simulink model "ccf"  (R2015b)
settings: Solver=VariableStepAuto  StartTime=0.0  StopTime=10.0  RelTol=1e-3
values from neighbouring files (symbols this model uses):
  Fx = inv((C*inv(-Ar)*B(:,1)))    [untitled.m]
settings Model: Creator=ovi  LastModifiedBy=ovi

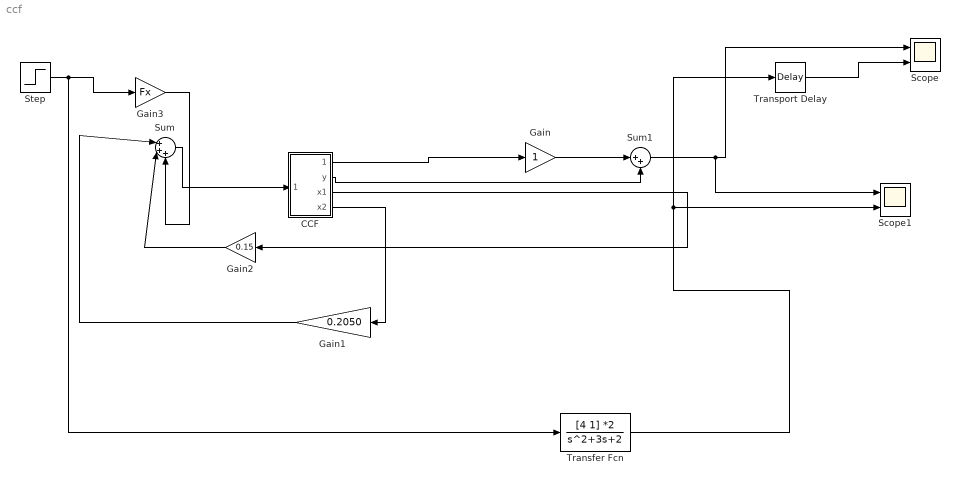
== system ccf ==
  CCF : Subsystem
  Gain : Gain
  Gain1 : Gain  Gain=0.2050
  Gain2 : Gain  Gain=0.15
  Gain3 : Gain  Gain=Fx
  Scope : Scope  NumInputPorts=2
  Scope1 : Scope  NumInputPorts=2
  Step : Step  SampleTime=0
  Sum : Sum  Inputs=|+++
  Sum1 : Sum  Inputs=|++
  Transfer Fcn : TransferFcn  Numerator=[4 1] *2  Denominator=[1 3 2]
  Transport Delay : TransportDelay  DelayTime=0.1
  wires:
  Gain/1 -> Sum1/1
  Sum1/1 -> Scope1/1, Scope/1
  CCF/1(Out1) -> Gain/1
  CCF/2(y) -> Sum1/2
  Transfer Fcn/1 -> Scope1/2, Transport Delay/1
  Transport Delay/1 -> Scope/2
  CCF/3("x1 ") -> Gain2/1
  CCF/4(x2) -> Gain1/1
  Gain2/1 -> Sum/2
  Gain1/1 -> Sum/1
  Step/1 -> Transfer Fcn/1, Gain3/1
  Gain3/1 -> Sum/3
  Sum/1 -> CCF/1(In1)

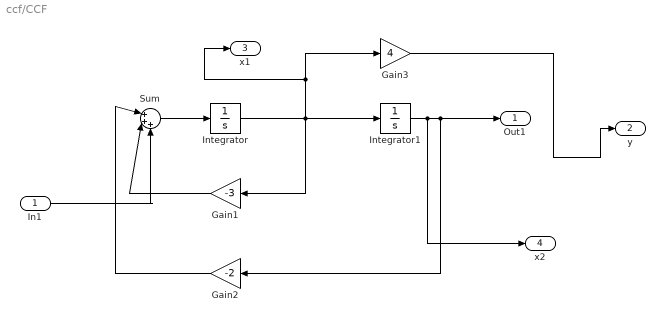
== system ccf/CCF ==
  In1 : Inport
  Gain1 : Gain  Gain=-3
  Gain2 : Gain  Gain=-2
  Gain3 : Gain  Gain=4
  Integrator : Integrator
  Integrator1 : Integrator
  Sum : Sum  Inputs=|+++
  Out1 : Outport
  y : Outport  Port=2
  "x1 " : Outport  Port=3
  x2 : Outport  Port=4
  wires:
  Gain3/1 -> y/1
  Integrator/1 -> Gain3/1, "x1 "/1, Gain1/1, Integrator1/1
  In1/1 -> Sum/3
  Gain1/1 -> Sum/2
  Integrator1/1 -> x2/1, Out1/1, Gain2/1
  Gain2/1 -> Sum/1
  Sum/1 -> Integrator/1
